simulink subsystem "CAS_PI_slash_D_Controller"  (R2024a)
settings: Solver=VariableStepAuto  StartTime=0.0  StopTime=10.0  RelTol=1e-3
values from neighbouring files (symbols this model uses):
  Kdrr = 0.004    [Init_FLIGHT_Hexacopter_fromNCMS.m]
  Kirr = 0.0    (= 0)    [Init_FLIGHT_Hexacopter_fromNCMS.m]
  Kprr = 0.1    [Init_FLIGHT_Hexacopter_fromNCMS.m]
  Nrr = 50    [Init_FLIGHT_Hexacopter_fromNCMS.m]
  SampleTime = 1/250    (= 0.004)    [Init_FLIGHT_Hexacopter.m]    (also in Init_FLIGHT_Hexacopter_fromNCMS.m = 0.01)
libraries: simulink x1, cstblocks x1, slpidlib x1
settings Model: Creator=sslee  LastModifiedBy=sslee

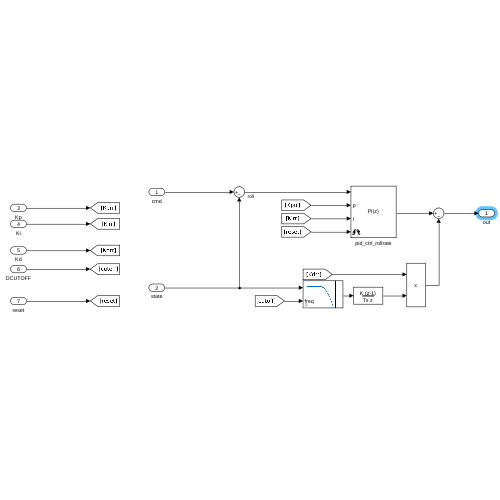
[thumbnail: Simulink's stored preview of the top-level diagram]
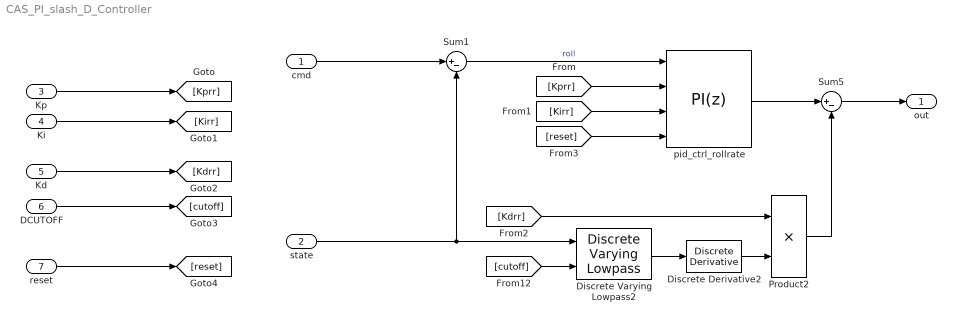
== system CAS_PI_slash_D_Controller ==
  cmd : Inport
  state : Inport  Port=2
  Kp : Inport  Port=3
  Ki : Inport  Port=4
  Kd : Inport  Port=5
  DCUTOFF : Inport  Port=6
  reset : Inport  Port=7
  Discrete Derivative2 : simulink/Discrete/Discrete Derivative  gainval=1.0  ICPrevScaledInput=0.0  OutMin=[]  OutMax=[]  OutDataType=fixdt(1, 16)  OutScaling=2^-10  DoSatur=off
  Discrete Varying Lowpass2 : cstblocks/Linear Parameter Varying/Discrete Varying Lowpass  N=2  w0=0  Ts=SampleTime
  Product2 : Product
  Sum1 : Sum  Inputs=|+-
  Sum5 : Sum  Inputs=|+-
  pid_ctrl_rollrate : slpidlib/PID Controller  Controller=PI  Form=Parallel  TimeDomain=Discrete-time  UseExternalTs=off  SampleTime=SampleTime  IntegratorMethod=Forward Euler  FilterMethod=Forward Euler  ControllerParametersSource=external  P=Kprr  I=Kirr  UseKiTs=off  D=Kdrr  UseExternalDerivativeSource=off  N=Nrr  UseFilter=on  TunerSelectOption=Transfer Function Based (PID Tuner App)  InitialConditionSource=internal  InitialConditionForIntegrator=0  InitialConditionForFilter=0  DifferentiatorICPrevScaledInput=0  ExternalReset=either  TrackingMode=off  Kt=1  LimitOutput=off  SatLimitsSource=internal  UpperSaturationLimit=0.2  LowerSaturationLimit=-0.2  LinearizeAsGain=on  AntiWindupMode=clamping  Kb=1  LimitIntegrator=off  UpperIntegratorSaturationLimit=inf  LowerIntegratorSaturationLimit=-inf  SaturateOnIntegerOverflow=on  POutMin=[]  POutMax=[]  IOutMin=[]  IOutMax=[]  DOutMin=[]  DOutMax=[]  NOutMin=[]  NOutMax=[]  SumOutMin=[]  SumOutMax=[]  SaturationOutDataTypeStr=single  SaturationOutMin=[]  SaturationOutMax=[]  PParamMin=[]  PParamMax=[]  IParamMin=[]  IParamMax=[]  DParamMin=[]  DParamMax=[]  NParamMin=[]  NParamMax=[]  KbParamMin=[]  KbParamMax=[]  KtParamMin=[]  KtParamMax=[]  KbOutMin=[]  KbOutMax=[]  KtOutMin=[]  KtOutMax=[]  IntegratorOutMin=[]  IntegratorOutMax=[]  FilterOutMin=[]  FilterOutMax=[]  SumI1OutMin=[]  SumI1OutMax=[]  SumI2OutMin=[]  SumI2OutMax=[]  SumI3OutMin=[]  SumI3OutMax=[]  SumI4OutMin=[]  SumI4OutMax=[]  SumDOutMin=[]  SumDOutMax=[]  DifferentiatorOutMin=[]  DifferentiatorOutMax=[]  FilterDiffOutCoefMin=[]  FilterDiffOutCoefMax=[]  ReciprocalOutMin=[]  ReciprocalOutMax=[]  SumDenOutMin=[]  SumDenOutMax=[]  SumNumOutMin=[]  SumNumOutMax=[]  DivideOutMin=[]  DivideOutMax=[]  UdiffTsProdOutMin=[]  UdiffTsProdOutMax=[]  NTsProdOutMin=[]  NTsProdOutMax=[]  UintegralTsProdOutMin=[]  UintegralTsProdOutMax=[]  UngainTsProdOutMin=[]  UngainTsProdOutMax=[]  ClampingZeroOutDataTypeStr=Inherit: Inherit via back propagation  ClampingZeroOutMin=[]  ClampingZeroOutMax=[]  FilterDenConstantOutDataTypeStr=Inherit: Inherit via back propagation  FilterDenConstantOutMin=[]  FilterDenConstantOutMax=[]  PCopyOutDataTypeStr=Inherit: Inherit via back propagation  PCopyOutMin=[]  PCopyOutMax=[]  NCopyOutDataTypeStr=Inherit: Inherit via back propagation  NCopyOutMin=[]  NCopyOutMax=[]  IntegratorContinuousStateAttributes=''  IntegratorStateMustResolveToSignalObject=off  IntegratorRTWStateStorageClass=Auto  FilterContinuousStateAttributes=''  FilterStateMustResolveToSignalObject=off  FilterRTWStateStorageClass=Auto  ParallelPVariant=ExternalParameters  IdealPVariant=Disabled  IVariant=ExternalParameters  DVariant=Disabled  IntegratorVariant=Discrete  SatVariant=Disabled  AWVariant=Passthrough  PCopyVariant=Disabled  TRVariant=Disabled  FdbkBlocksVariant=Forward  IdealPFdbkVariant=Disabled  SatFdbkVariant=Disabled  DerivativeFilterVariant=Disabled  NVariant=Disabled  NCopyVariant=Disabled_SignalSpec  FilterICVariant=Disabled  IntegratorICVariant=InternalICs  ExternalResetVariant=ExternalReset  TRSumVariant=Passthrough  SumFdbkVariant=Disabled  SumVariant=Sum_PI  TsampFilterVariant=InternalTs  TsampNgainVariant=Passthrough  TsampIntegralVariant=Disabled_SignalSpec  ExternalSaturationOutDataTypeStr=single  DerivativeSourceVariant=Disabled
  out : Outport
  wires:
  Sum1/1 -> pid_ctrl_rollrate/1  "roll"
  [Kirr] -> pid_ctrl_rollrate/3
  [cutoff] -> Discrete Varying Lowpass2/2
  Product2/1 -> Sum5/2
  Discrete Varying Lowpass2/1 -> Discrete Derivative2/1
  Discrete Derivative2/1 -> Product2/2
  Sum5/1 -> out/1
  [Kprr] -> pid_ctrl_rollrate/2
  [Kdrr] -> Product2/1
  pid_ctrl_rollrate/1 -> Sum5/1
  Kp/1 -> [Kprr]
  Ki/1 -> [Kirr]
  Kd/1 -> [Kdrr]
  DCUTOFF/1 -> [cutoff]
  state/1 -> Sum1/2, Discrete Varying Lowpass2/1
  reset/1 -> [reset]
  [reset] -> pid_ctrl_rollrate/4
  cmd/1 -> Sum1/1
